simulink model "MRAC_SISO"  (R2015b)
settings: Solver=VariableStepAuto  StartTime=0.0  StopTime=40  RelTol=1e-3
settings Model: Creator=admin  LastModifiedBy=admin

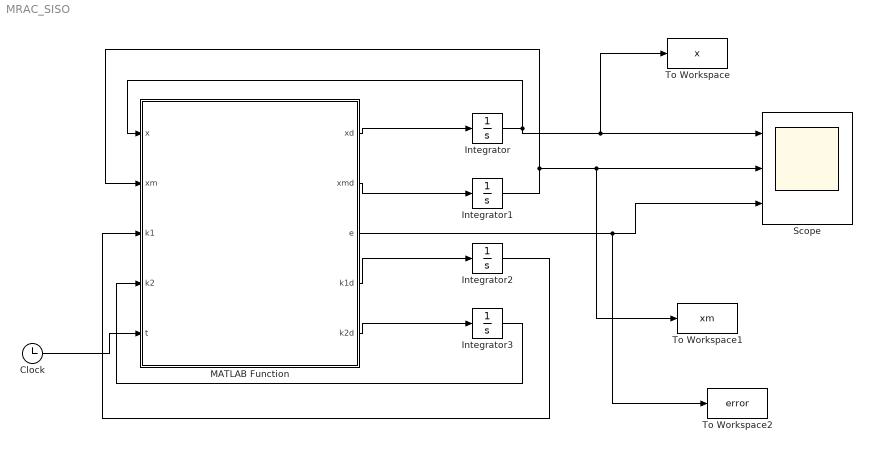
== system MRAC_SISO ==
  Clock : Clock
  Integrator{,1..3} (4 alike) : Integrator
  MATLAB Function : MATLAB Function  TreatAsAtomicUnit=on
  Scope : Scope  NumInputPorts=3
  To Workspace : ToWorkspace  VariableName=x  SaveFormat=Timeseries  SampleTime=-1
  To Workspace1 : ToWorkspace  VariableName=xm  SaveFormat=Timeseries  SampleTime=-1
  To Workspace2 : ToWorkspace  VariableName=error  SaveFormat=Timeseries  SampleTime=-1
  wires:
  MATLAB Function/1(xd) -> Integrator/1
  MATLAB Function/2(xmd) -> Integrator1/1
  MATLAB Function/4(k1d) -> Integrator2/1
  MATLAB Function/5(k2d) -> Integrator3/1
  Integrator/1 -> MATLAB Function/1(x), To Workspace/1, Scope/1
  Integrator1/1 -> To Workspace1/1, Scope/2, MATLAB Function/2(xm)
  Integrator3/1 -> MATLAB Function/4(k2)
  Integrator2/1 -> MATLAB Function/3(k1)
  MATLAB Function/3(e) -> To Workspace2/1, Scope/3
  Clock/1 -> MATLAB Function/5(t)

== matlab function MRAC_SISO/MATLAB Function ==
  data: x input; xm input; xd output; k1 input; k2 input; xmd output; e output; k1d output; k2d output; t input
function [xd,xmd,e,k1d,k2d] = fcn(x,xm,k1,k2,t)
e=x-xm;
r=(1-exp(-2*t));

%% Controller
u=k1*x+k2*r;


%% system model
a=-2;
b=-2;
xd=a*x+b*u;

%% Reference model
am=-3;
bm=2
xmd=am*xm+bm*r;
%% Controller parameter update law
%P=[1/4 0;0 1/6];
gamma1=10;%[1 0;0 1];
gamma2=10;%[1 0;0 1];
k1d=-gamma1*x*e*sign(b);
k2d=-gamma2*r*e*sign(b);
